simulink library "ElectricConsumptionPump"  (R2018b)
settings: Solver=ode45  StartTime=0.0  StopTime=10.0  RelTol=1e-3  EnableMultiTasking=on
libraries: simulink x1
settings Model: Creator=lena.frank  LastModifiedBy=P41573
settings DataIOCC: LimitDataPoints=on  SaveFormat=Array  SignalLoggingSaveFormat=ModelDataLogs
settings OptimizationCC: ExpressionDepthLimit=2147483647  LifeSpan=inf
settings DebuggingCC: UnderspecifiedInitializationDetection=Classic  MergeDetectMultiDrivingBlocksExec=none  SolverPrmCheckMsg=warning  FcnCallInpInsideContextMsg=warning  StateNameClashWarn=warning  SFUnexpectedBacktrackingDiag=warning  SFNoUnconditionalDefaultTransitionDiag=warning  SFExecutionAtInitializationDiag=none
settings HardwareCC: ProdBitPerPointer=32  ProdBitPerSizeT=32  ProdBitPerPtrDiffT=32  ProdLargestAtomicFloat=None  ProdIntDivRoundTo=Undefined  ProdEndianess=Unspecified  ProdWordSize=32  ProdHWDeviceType=32-bit Generic
settings ModelReferenceCC: PropagateSignalLabelsOutOfModel=off
settings SFSimCC: SimUseLocalCustomCode=off
settings RTWCC: RTWUseLocalCustomCode=off
settings CodeAppCC: StateflowObjectComments=on
settings GRTTargetCC: TargetLangStandard=C89/C90 (ANSI)  GeneratePreprocessorConditionals=Disable all  CombineOutputUpdateFcns=off  GRTInterface=on
settings ConfigComp: CovMetricSettings=dw  CovHtmlReporting=on  CovSaveCumulativeToWorkspaceVar=on  CovSaveSingleToWorkspaceVar=on  CovExternalEMLEnable=off

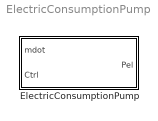
== system ElectricConsumptionPump ==
  ElectricConsumptionPump : Subsystem  mask(Electric Consumption of a Pump){e0=10, e1=10, e2=-1}
      mask prompts: e0 "e0: constant coefficient in W"; e1 "e1: linear coefficient in W*s/kg"; e2 "e2: quadratic coefficient in W*(s/kg)²"
      mask help:
      | The electric consumption of the pump is given by the quadratic equation
      |   Pel = e0 + e1*mdot + e2*mdot^2
      | with
      |   mdot : massflow in kg/s
      |   Pel : electric consumption in W
      mask TypeOptions e0: Constant/Value
      mask TypeOptions e1: Linear/Gain
      mask TypeOptions e2: Quadratic/Gain
      mask Display: disp('Pel = e0\n+ e1*mdot\n+ e2*mdot² ')

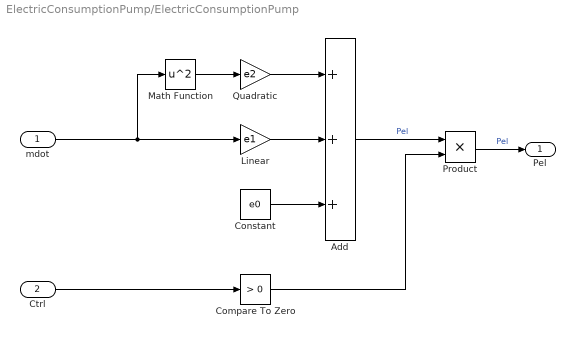
== system ElectricConsumptionPump/ElectricConsumptionPump ==
  mdot : Inport
  Ctrl : Inport  Port=2
  Add : Sum  Inputs=3
  Compare To Zero : simulink/Logic and Bit Operations/Compare To Zero  relop=>  OutDataTypeStr=boolean
  Constant : Constant  Value=e0
  Linear : Gain  Gain=e1
  Math Function : Math  Operator=square  SaturateOnIntegerOverflow=on
  Product : Product
  Quadratic : Gain  Gain=e2
  Pel : Outport
  wires:
  Quadratic/1 -> Add/1
  mdot/1 -> Linear/1, Math Function/1
  Linear/1 -> Add/2
  Math Function/1 -> Quadratic/1
  Product/1 -> Pel/1  "Pel"
  Constant/1 -> Add/3
  Ctrl/1 -> Compare To Zero/1
  Add/1 -> Product/1  "Pel"
  Compare To Zero/1 -> Product/2
